simulink subsystem "GravityTorque"  (R2021a)
settings: Solver=VariableStepAuto  StartTime=0.0  StopTime=10.0  RelTol=1e-3
undefined symbols (not defined in the file): Ix, Iy, Iz, mu
libraries: aerolibutil x1
settings Model: Creator=Laura  LastModifiedBy=Laura

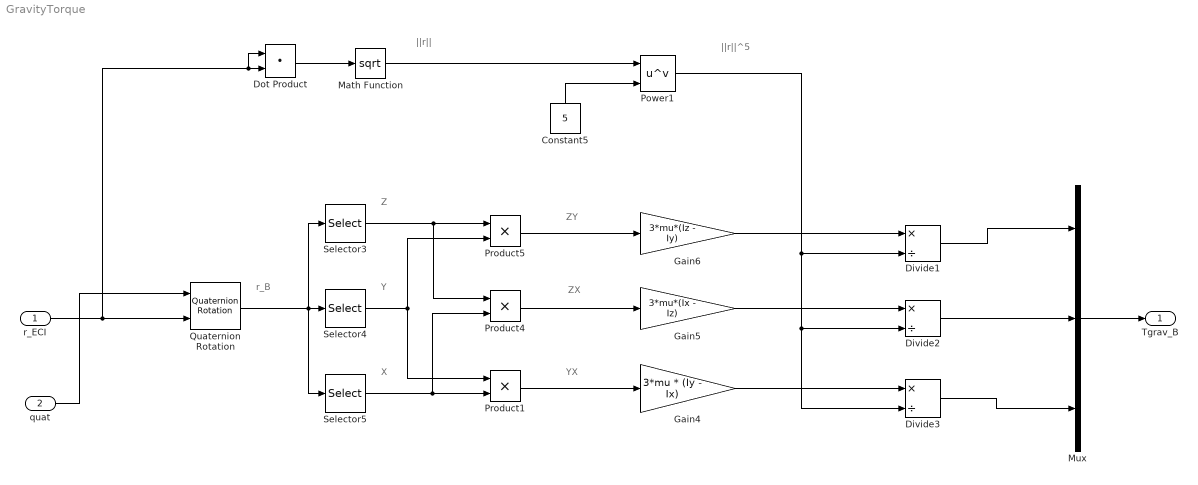
== system GravityTorque ==
  note: r_B
  note: X
  note: ZX
  note: Y
  note: YX
  note: ||r||^5
  note: Z
  note: ZY
  note: ||r||
  r_ECI : Inport
  quat : Inport  Port=2
  Constant5 : Constant  Value=5
  Divide1 : Product  Inputs=*/
  Divide2 : Product  Inputs=*/
  Divide3 : Product  Inputs=*/
  Dot Product : DotProduct  InputSameDT=on  OutDataTypeStr=Inherit: Inherit via internal rule
  Gain4 : Gain  Gain=3*mu * (Iy - Ix)
  Gain5 : Gain  Gain=3*mu*(Ix - Iz)
  Gain6 : Gain  Gain=3*mu*(Iz - Iy)
  Math Function : Math  Operator=sqrt  SignedPower=on  SaturateOnIntegerOverflow=on
  Mux : Mux  Inputs=3
  Power1 : Math  Operator=pow  SaturateOnIntegerOverflow=on
  Product1 : Product
  Product4 : Product
  Product5 : Product
  Quaternion Rotation : aerolibutil/Quaternion Rotation
  Selector3 : Selector  InputPortWidth=3  IndexOptions=Index vector (dialog)  Indices=[3]  OutputSizes=1
  Selector4 : Selector  InputPortWidth=3  IndexOptions=Index vector (dialog)  Indices=[2]  OutputSizes=1
  Selector5 : Selector  InputPortWidth=3  IndexOptions=Index vector (dialog)  Indices=[1]  OutputSizes=1
  Tgrav_B : Outport
  wires:
  Gain6/1 -> Divide1/1
  Product5/1 -> Gain6/1
  Constant5/1 -> Power1/2
  Selector4/1 -> Product1/1, Product5/2
  Selector3/1 -> Product4/1, Product5/1
  Selector5/1 -> Product1/2, Product4/2
  Gain4/1 -> Divide3/1
  Quaternion Rotation/1 -> Selector5/1, Selector3/1, Selector4/1
  Gain5/1 -> Divide2/1
  Product4/1 -> Gain5/1
  Product1/1 -> Gain4/1
  Dot Product/1 -> Math Function/1
  Math Function/1 -> Power1/1
  Power1/1 -> Divide3/2, Divide2/2, Divide1/2
  Divide1/1 -> Mux/1
  Divide2/1 -> Mux/2
  Divide3/1 -> Mux/3
  Mux/1 -> Tgrav_B/1
  r_ECI/1 -> Dot Product/2, Dot Product/1, Quaternion Rotation/2
  quat/1 -> Quaternion Rotation/1
